simulink model "cascadeControl"  (R2020b)
settings: Solver=VariableStepAuto  StartTime=0.0  StopTime=40  RelTol=1e-3
values from neighbouring files (symbols this model uses):
  a_max = 4    [initialization.m]
  condtheta = 0    [initialization.m]
  condx = 0.0001    [initialization.m]
  condy = 0    [initialization.m]
  k = 1    [initialization.m]
  k_a = 2    [initialization.m]
  k_obsx = 5    [initialization.m]
  k_obsy = 5    [initialization.m]
  omega_max = 0.1    [initialization.m]
  slope_circ = 0.2    [initialization.m]
  v_max = 0.5    [initialization.m]
  v_square = 0.2    [initialization.m]
undefined symbols (not defined in the file or in its folder): sat_om
libraries: simulink x2
settings Model: Creator=adelina  LastModifiedBy=adelina
settings SolverCC: ZeroCrossAlgorithm=Adaptive
settings DebuggingCC: IgnoredZcDiagnostic=none

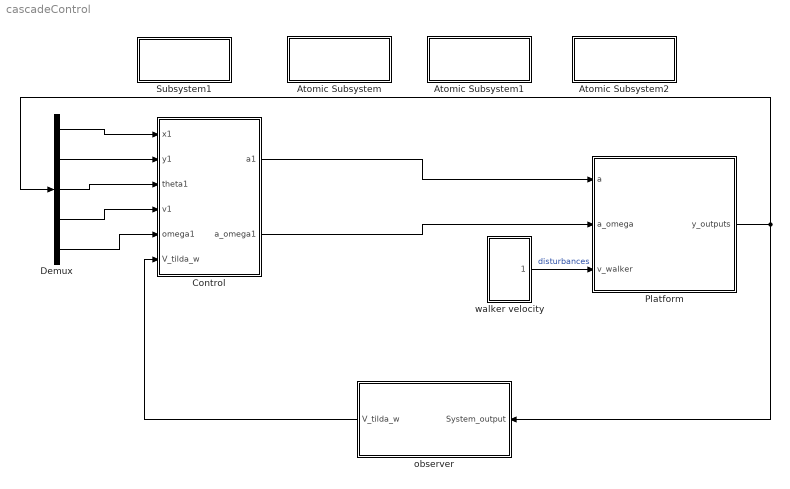
== system cascadeControl ==
  Atomic Subsystem : Subsystem  TreatAsAtomicUnit=on
      settings: OpenFcn=animation
      mask Display: disp('animation')
  Atomic Subsystem1 : Subsystem  TreatAsAtomicUnit=on
      settings: OpenFcn=plot_inputs
      mask Display: disp('plot inputs')
  Atomic Subsystem2 : Subsystem  TreatAsAtomicUnit=on
      settings: OpenFcn=plot_states
      mask Display: disp('plot states')
  Control : Subsystem
  Demux : Demux  Outputs=5
  Platform : Subsystem
  Subsystem1 : Subsystem
      settings: OpenFcn=plot_trajectory_frames
      mask Display: disp('plots')
  observer : Subsystem
  walker velocity : Subsystem
  wires:
  walker velocity/1(v_walker) -> Platform/3(v_walker)  "disturbances"
  Platform/1(y_outputs) -> observer/1(System_output), Demux/1
  Control/1(a1) -> Platform/1(a)
  Control/2(a_omega1) -> Platform/2(a_omega)
  Demux/3 -> Control/3(theta1)
  Demux/2 -> Control/2(y1)
  Demux/1 -> Control/1(x1)
  Demux/4 -> Control/4(v1)
  Demux/5 -> Control/5(omega1)
  observer/1(V_tilda_w) -> Control/6(V_tilda_w)

== system cascadeControl/Atomic Subsystem ==

== system cascadeControl/Atomic Subsystem1 ==

== system cascadeControl/Atomic Subsystem2 ==

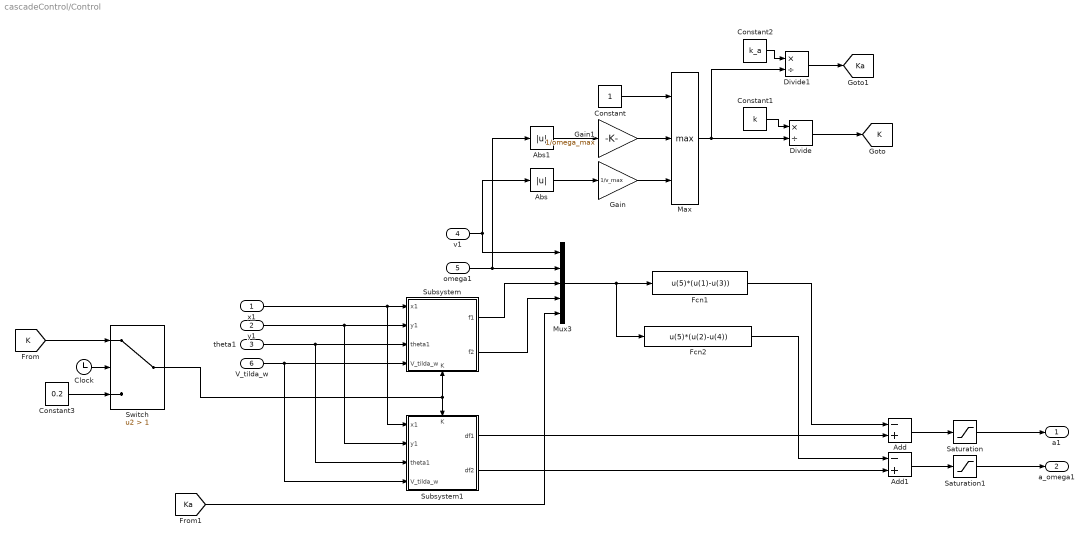
== system cascadeControl/Control ==
  x1 : Inport
  y1 : Inport  Port=2
  theta1 : Inport  Port=3
  v1 : Inport  Port=4
  omega1 : Inport  Port=5
  V_tilda_w : Inport  Port=6
  Abs : Abs
  Abs1 : Abs
  Add : Sum  Inputs=-+
  Add1 : Sum  Inputs=-+
  Clock : Clock
  Constant : Constant
  Constant1 : Constant  Value=k
  Constant2 : Constant  Value=k_a
  Constant3 : Constant  Value=0.2
  Divide : Product  Inputs=*/  RndMeth=Zero  SaturateOnIntegerOverflow=on
  Divide1 : Product  Inputs=*/  RndMeth=Zero  SaturateOnIntegerOverflow=on
  Fcn1 : Fcn  Expr=u(5)*(u(1)-u(3))
  Fcn2 : Fcn  Expr=u(5)*(u(2)-u(4))
  Gain : Gain  Gain=1/v_max
  Gain1 : Gain  Gain=1/omega_max
  Max : MinMax  Function=max  Inputs=3
  Mux3 : Mux  Inputs=5
  Saturation : Saturate  UpperLimit=a_max  LowerLimit=-a_max  ZeroCross=off
  Saturation1 : Saturate  UpperLimit=a_max  LowerLimit=-a_max  ZeroCross=off
  Subsystem : Subsystem
      settings: PortSchema="{\"entries\":[{\"content\":{\"sides\":[{\"content\":{\"connectorIds\":[\"In1\",\"In2\",\"In3\",\"In4\"]},\"type\":\"ConnectorPlacement.EquallySpacedRectSide\",\"uuid\":\"98a92254-b9ad-4bc0-80a4-de031a5e2866\"},{\"content\":{\"connectorIds\":[\"Out1\",\"Out2\"],\"side\":\"RIGHT\"},\"type\":\"ConnectorPlacement.EquallySpacedRectSide\",\"uuid\":\"e0692c06-8f6c-4190-87dc-563178f83e51\"},{\"content\":{\"connectorIds\":[],\"side\":\"TOP\"},\"type\":\"ConnectorPlacement.EquallySpacedRectSide\",\"uuid\":\"24e54c67-c633-4464-84bd-e02cec2cb8a7\"},{\"content\":{\"connectorIds\":[\"In5\"],\"side\":\"BOTTOM\"},\"type\":\"ConnectorPlacement.EquallySpacedRectSide\",\"uuid\":\"19ff3774-67e6-4579-b3b2-94cf61eef82b\"},{\"content\":{\"connectorIds\":[],\"side\":\"HIDDEN\"},\"type\":\"ConnectorPlacement.EquallySpacedRectSide\",\"uuid\":\"6a6977b6-e148-496e-85eb-1bd9ad7285df\"}]},\"type\":\"ConnectorPlacement.EquallySpacedConnector\",\"uuid\":\"5663e86b-5163-4af1-b1c3-40fc09afe5cc\"}],\"packageUris\":[\"http://schema.mathworks.com/mf0/Connector/R2020b\"],\"version\":\"1.0\"}"
  Subsystem1 : Subsystem
      settings: PortSchema="{\"entries\":[{\"content\":{\"sides\":[{\"content\":{\"connectorIds\":[\"In1\",\"In2\",\"In3\",\"In4\"]},\"type\":\"ConnectorPlacement.EquallySpacedRectSide\",\"uuid\":\"98a92254-b9ad-4bc0-80a4-de031a5e2866\"},{\"content\":{\"connectorIds\":[\"Out1\",\"Out2\"],\"side\":\"RIGHT\"},\"type\":\"ConnectorPlacement.EquallySpacedRectSide\",\"uuid\":\"e0692c06-8f6c-4190-87dc-563178f83e51\"},{\"content\":{\"connectorIds\":[\"In5\"],\"side\":\"TOP\"},\"type\":\"ConnectorPlacement.EquallySpacedRectSide\",\"uuid\":\"24e54c67-c633-4464-84bd-e02cec2cb8a7\"},{\"content\":{\"connectorIds\":[],\"side\":\"HIDDEN\"},\"type\":\"ConnectorPlacement.EquallySpacedRectSide\",\"uuid\":\"6a6977b6-e148-496e-85eb-1bd9ad7285df\"}]},\"type\":\"ConnectorPlacement.EquallySpacedConnector\",\"uuid\":\"5663e86b-5163-4af1-b1c3-40fc09afe5cc\"}],\"packageUris\":[\"http://schema.mathworks.com/mf0/Connector/R2020b\"],\"version\":\"1.0\"}"
  Switch : Switch  Criteria=u2 > Threshold  Threshold=1
  a1 : Outport
  a_omega1 : Outport  Port=2
  tag scope: K=global, Ka=global
  wires:
  x1/1 -> Subsystem1/1(x1), Subsystem/1(x1)
  y1/1 -> Subsystem1/2(y1), Subsystem/2(y1)
  theta1/1 -> Subsystem1/3(theta1), Subsystem/3(theta1)
  Subsystem/1(f1) -> Mux3/3
  Subsystem/2(f2) -> Mux3/4
  Mux3/1 -> Fcn1/1, Fcn2/1
  Subsystem1/1(df1) -> Add/2
  Fcn1/1 -> Add/1
  Fcn2/1 -> Add1/1
  Subsystem1/2(df2) -> Add1/2
  v1/1 -> Mux3/1, Abs/1
  omega1/1 -> Abs1/1, Mux3/2
  V_tilda_w/1 -> Subsystem1/4(V_tilda_w), Subsystem/4(V_tilda_w)
  Abs/1 -> Gain/1
  Gain/1 -> Max/3
  Abs1/1 -> Gain1/1
  Gain1/1 -> Max/2
  Constant/1 -> Max/1
  Max/1 -> Divide/2, Divide1/2
  Constant1/1 -> Divide/1
  Divide/1 -> [K]
  Saturation1/1 -> a_omega1/1
  Add1/1 -> Saturation1/1
  Add/1 -> Saturation/1
  Saturation/1 -> a1/1
  [Ka] -> Mux3/5
  Constant2/1 -> Divide1/1
  Divide1/1 -> [Ka]
  [K] -> Switch/1
  Clock/1 -> Switch/2
  Constant3/1 -> Switch/3
  Switch/1 -> Subsystem/5(K), Subsystem1/5(K)

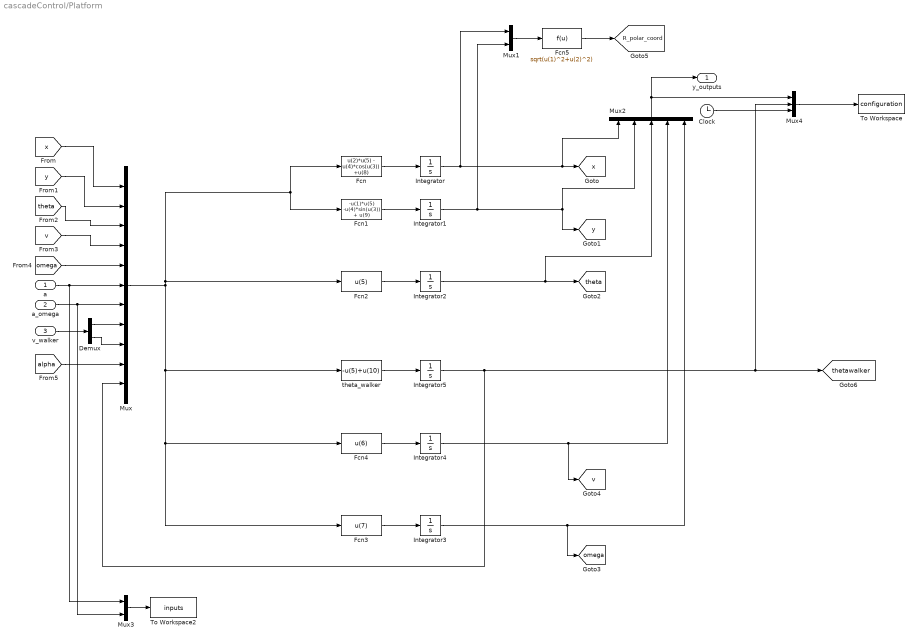
== system cascadeControl/Platform ==
  a : Inport
  a_omega : Inport  Port=2
  v_walker : Inport  Port=3
  Clock : Clock
  Demux : Demux  Outputs=2
  Fcn : Fcn  Expr=u(2)*u(5) - u(4)*cos(u(3)) +u(8)
  Fcn1 : Fcn  Expr=-u(1)*u(5) -u(4)*sin(u(3)) + u(9)
  Fcn2 : Fcn  Expr=u(5)
  Fcn3 : Fcn  Expr=u(7)
  Fcn4 : Fcn  Expr=u(6)
  Fcn5 : Fcn  Expr=sqrt(u(1)^2+u(2)^2)
  Integrator : Integrator  InitialCondition=condx
  Integrator1 : Integrator  InitialCondition=condy
  Integrator2 : Integrator  InitialCondition=condtheta
  Integrator3 : Integrator
  Integrator4 : Integrator
  Integrator5 : Integrator  InitialCondition=condtheta
  Mux : Mux  Inputs=11
  Mux1 : Mux  Inputs=2
  Mux2 : Mux  Inputs=5
  Mux3 : Mux  Inputs=2
  Mux4 : Mux  Inputs=3
  To Workspace : ToWorkspace  VariableName=configuration  SaveFormat=Structure With Time  SampleTime=-1
  To Workspace2 : ToWorkspace  VariableName=inputs  SaveFormat=Structure With Time  SampleTime=-1
  theta_walker : Fcn  Expr=-u(5)+u(10)
  y_outputs : Outport
  tag scope: R_polar_coord=global, omega=global, theta=global, thetawalker=global, v=global, x=global, y=global
  wires:
  Fcn2/1 -> Integrator2/1
  Integrator2/1 -> [theta], Mux2/3
  Fcn1/1 -> Integrator1/1
  [y] -> Mux/2
  [x] -> Mux/1
  a/1 -> Mux3/1, Mux/6
  Integrator1/1 -> Mux1/2, [y], Mux2/2
  [theta] -> Mux/3
  Integrator/1 -> Mux1/1, Mux2/1, [x]
  Fcn/1 -> Integrator/1
  a_omega/1 -> Mux3/2, Mux/7
  Mux2/1 -> y_outputs/1, Mux4/1
  [v] -> Mux/4
  [omega] -> Mux/5
  Integrator3/1 -> Mux2/5, [omega]
  Fcn3/1 -> Integrator3/1
  Integrator4/1 -> [v], Mux2/4
  Fcn4/1 -> Integrator4/1
  Mux1/1 -> Fcn5/1
  Fcn5/1 -> [R_polar_coord]
  Mux3/1 -> To Workspace2/1
  Clock/1 -> Mux4/3
  Mux4/1 -> To Workspace/1
  v_walker/1 -> Demux/1
  Demux/1 -> Mux/8
  Demux/2 -> Mux/9
  [alpha] -> Mux/10
  Mux/1 -> Fcn1/1, Fcn/1, Fcn2/1, theta_walker/1, Fcn3/1, Fcn4/1
  theta_walker/1 -> Integrator5/1
  Integrator5/1 -> Mux/11, [thetawalker], Mux4/2

== system cascadeControl/Subsystem1 ==

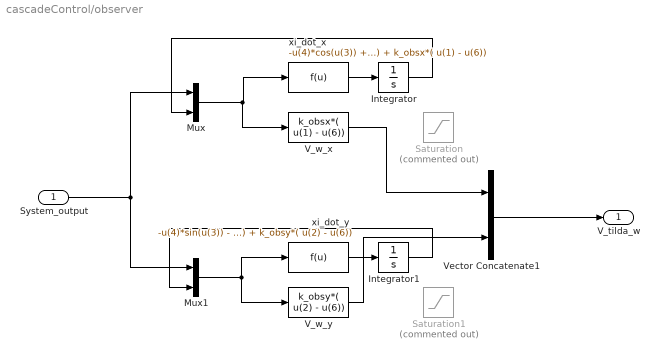
== system cascadeControl/observer ==
  System_output : Inport
  Integrator : Integrator  InitialCondition=condx
  Integrator1 : Integrator  InitialCondition=condy
  Mux : Mux  Inputs=2
  Mux1 : Mux  Inputs=2
  Saturation : Saturate  Commented=on
  Saturation1 : Saturate  Commented=on
  V_w_x : Fcn  Expr=k_obsx*( u(1) - u(6))
  V_w_y : Fcn  Expr=k_obsy*( u(2) - u(6))
  Vector Concatenate1 : Concatenate  Mode=Multidimensional array  ConcatenateDimension=2
  xi_dot_x : Fcn  Expr=-u(4)*cos(u(3)) + u(2)*u(5) + k_obsx*( u(1) - u(6))
  xi_dot_y : Fcn  Expr=-u(4)*sin(u(3)) - u(1)*u(5) + k_obsy*( u(2) - u(6))
  V_tilda_w : Outport
  wires:
  Mux/1 -> V_w_x/1, xi_dot_x/1
  Mux1/1 -> V_w_y/1, xi_dot_y/1
  System_output/1 -> Mux/1, Mux1/1
  Vector Concatenate1/1 -> V_tilda_w/1
  xi_dot_x/1 -> Integrator/1
  Integrator/1 -> Mux/2
  xi_dot_y/1 -> Integrator1/1
  Integrator1/1 -> Mux1/2
  V_w_y/1 -> Vector Concatenate1/2
  V_w_x/1 -> Vector Concatenate1/1

== system cascadeControl/walker velocity ==
  Circular path : Subsystem
  DocBlock : simulink/Model-Wide Utilities/DocBlock  DocumentType=Text
      content=|
      | Choose one of the trajectory by uncommenting and connecting with the output
  "Vx, Vy nonzero" : Subsystem  Commented=on
  square path : Subsystem  Commented=on
  v_walker : Outport
  wires:
  Circular path/1(v_walker) -> v_walker/1

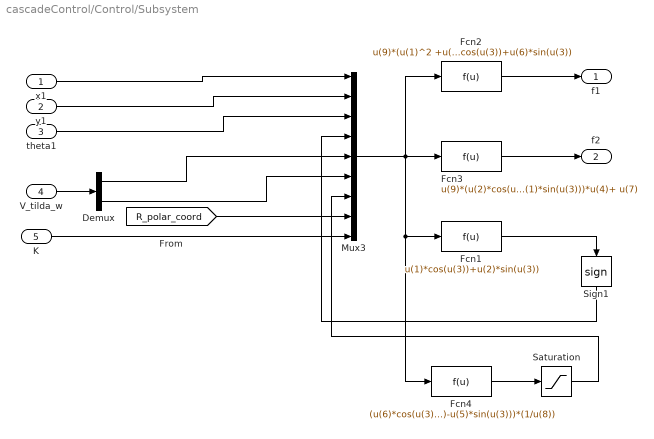
== system cascadeControl/Control/Subsystem ==
  x1 : Inport
  y1 : Inport  Port=2
  theta1 : Inport  Port=3
  V_tilda_w : Inport  Port=4
  K : Inport  Port=5
  Demux : Demux  Outputs=2
  Fcn1 : Fcn  Expr=u(1)*cos(u(3))+u(2)*sin(u(3))
  Fcn2 : Fcn  Expr=u(9)*(u(1)^2 +u(2)^2)*u(4)+u(5)*cos(u(3))+u(6)*sin(u(3))
  Fcn3 : Fcn  Expr=u(9)*(u(2)*cos(u(3))-u(1)*sin(u(3)))*u(4)+ u(7)
  Fcn4 : Fcn  Expr=(u(6)*cos(u(3))-u(5)*sin(u(3)))*(1/u(8))
  Mux3 : Mux  Inputs=9
  Saturation : Saturate  UpperLimit=sat_om  LowerLimit=-sat_om
  Sign1 : Signum  ZeroCross=off
  f1 : Outport
  f2 : Outport  Port=2
  wires:
  Sign1/1 -> Mux3/4
  y1/1 -> Mux3/2
  x1/1 -> Mux3/1
  theta1/1 -> Mux3/3
  Fcn1/1 -> Sign1/1
  Mux3/1 -> Fcn4/1, Fcn1/1, Fcn2/1, Fcn3/1
  Fcn2/1 -> f1/1
  Fcn3/1 -> f2/1
  V_tilda_w/1 -> Demux/1
  Demux/1 -> Mux3/5
  Demux/2 -> Mux3/6
  Fcn4/1 -> Saturation/1
  Saturation/1 -> Mux3/7
  [R_polar_coord] -> Mux3/8
  K/1 -> Mux3/9

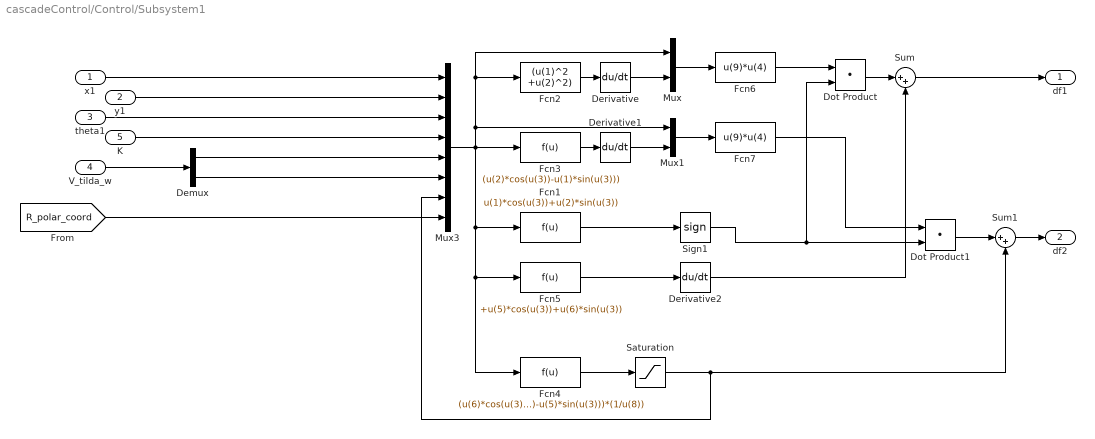
== system cascadeControl/Control/Subsystem1 ==
  x1 : Inport
  y1 : Inport  Port=2
  theta1 : Inport  Port=3
  V_tilda_w : Inport  Port=4
  K : Inport  Port=5
  Demux : Demux  Outputs=2
  Derivative : Derivative
  Derivative1 : Derivative
  Derivative2 : Derivative
  Dot Product : DotProduct  InputSameDT=on  OutDataTypeStr=Inherit: Inherit via internal rule
  Dot Product1 : DotProduct  InputSameDT=on  OutDataTypeStr=Inherit: Inherit via internal rule
  Fcn1 : Fcn  Expr=u(1)*cos(u(3))+u(2)*sin(u(3))
  Fcn2 : Fcn  Expr=(u(1)^2 +u(2)^2)
  Fcn3 : Fcn  Expr=(u(2)*cos(u(3))-u(1)*sin(u(3)))
  Fcn4 : Fcn  Expr=(u(6)*cos(u(3))-u(5)*sin(u(3)))*(1/u(8))
  Fcn5 : Fcn  Expr=+u(5)*cos(u(3))+u(6)*sin(u(3))
  Fcn6 : Fcn  Expr=u(9)*u(4)
  Fcn7 : Fcn  Expr=u(9)*u(4)
  Mux : Mux  Inputs=2
  Mux1 : Mux  Inputs=2
  Mux3 : Mux  Inputs=8
  Saturation : Saturate  UpperLimit=sat_om  LowerLimit=-sat_om
  Sign1 : Signum  ZeroCross=off
  Sum : Sum  Inputs=|++
  Sum1 : Sum  Inputs=|++
  df1 : Outport
  df2 : Outport  Port=2
  wires:
  y1/1 -> Mux3/2
  Fcn1/1 -> Sign1/1
  Mux3/1 -> Fcn3/1, Fcn1/1, Fcn5/1, Fcn4/1, Mux1/1, Fcn2/1, Mux/1
  theta1/1 -> Mux3/3
  Demux/1 -> Mux3/5
  x1/1 -> Mux3/1
  [R_polar_coord] -> Mux3/8
  Fcn4/1 -> Saturation/1
  Saturation/1 -> Sum1/2, Mux3/7
  V_tilda_w/1 -> Demux/1
  Demux/2 -> Mux3/6
  Fcn2/1 -> Derivative/1
  Fcn3/1 -> Derivative1/1
  Dot Product/1 -> Sum/1
  Fcn5/1 -> Derivative2/1
  Sum/1 -> df1/1
  Sum1/1 -> df2/1
  Derivative2/1 -> Sum/2
  Dot Product1/1 -> Sum1/1
  Sign1/1 -> Dot Product/2, Dot Product1/2
  K/1 -> Mux3/4
  Derivative/1 -> Mux/2
  Mux/1 -> Fcn6/1
  Fcn6/1 -> Dot Product/1
  Mux1/1 -> Fcn7/1
  Derivative1/1 -> Mux1/2
  Fcn7/1 -> Dot Product1/1

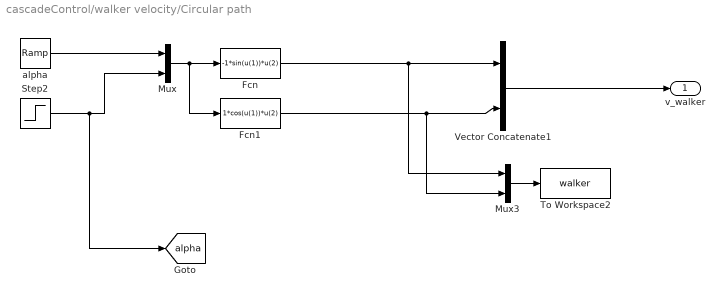
== system cascadeControl/walker velocity/Circular path ==
  Fcn : Fcn  Expr=-1*sin(u(1))*u(2)
  Fcn1 : Fcn  Expr=1*cos(u(1))*u(2)
  Mux : Mux  Inputs=2
  Mux3 : Mux  Inputs=2
  Step2 : Step  After=slope_circ  SampleTime=0
  To Workspace2 : ToWorkspace  VariableName=walker  SaveFormat=Structure With Time  SampleTime=-1
  Vector Concatenate1 : Concatenate  Mode=Multidimensional array  ConcatenateDimension=2
  alpha : simulink/Sources/Ramp  slope=slope_circ  start=1  InitialOutput=0
  v_walker : Outport
  tag scope: alpha=global
  wires:
  alpha/1 -> Mux/1
  Fcn1/1 -> Vector Concatenate1/2, Mux3/2
  Fcn/1 -> Mux3/1, Vector Concatenate1/1
  Vector Concatenate1/1 -> v_walker/1
  Mux3/1 -> To Workspace2/1
  Mux/1 -> Fcn1/1, Fcn/1
  Step2/1 -> [alpha], Mux/2

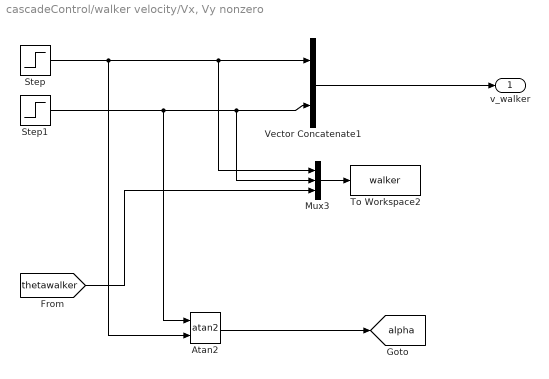
== system cascadeControl/walker velocity/Vx, Vy nonzero ==
  Atan2 : Trigonometry  Operator=atan2
  Mux3 : Mux  Inputs=3
  Step : Step  Time=2  After=0  SampleTime=0
  Step1 : Step  Time=0  After=0  SampleTime=0
  To Workspace2 : ToWorkspace  VariableName=walker  SaveFormat=Structure With Time  SampleTime=-1
  Vector Concatenate1 : Concatenate  Mode=Multidimensional array  ConcatenateDimension=2
  v_walker : Outport
  tag scope: alpha=global
  wires:
  Vector Concatenate1/1 -> v_walker/1
  Mux3/1 -> To Workspace2/1
  Step/1 -> Atan2/2, Mux3/1, Vector Concatenate1/1
  Step1/1 -> Atan2/1, Vector Concatenate1/2, Mux3/2
  [thetawalker] -> Mux3/3
  Atan2/1 -> [alpha]

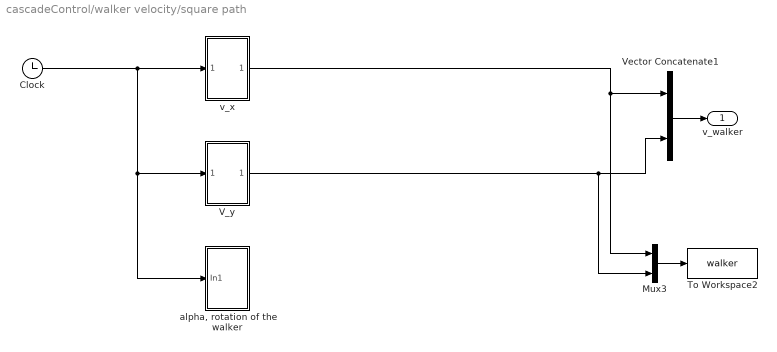
== system cascadeControl/walker velocity/square path ==
  Clock : Clock
  Mux3 : Mux  Inputs=2
  To Workspace2 : ToWorkspace  VariableName=walker  SaveFormat=Structure With Time  SampleTime=-1
  V_y : Subsystem
  Vector Concatenate1 : Concatenate  Mode=Multidimensional array  ConcatenateDimension=2
  "alpha, rotation of the walker" : Subsystem
  v_x : Subsystem
  v_walker : Outport
  wires:
  Vector Concatenate1/1 -> v_walker/1
  Mux3/1 -> To Workspace2/1
  Clock/1 -> v_x/1(In1), "alpha, rotation of the walker"/1(In1), V_y/1(In1)
  V_y/1(Out1) -> Mux3/2, Vector Concatenate1/2
  v_x/1(Out1) -> Mux3/1, Vector Concatenate1/1

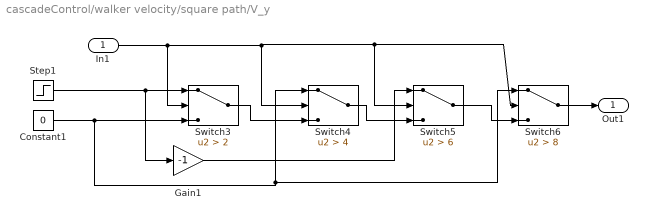
== system cascadeControl/walker velocity/square path/V_y ==
  In1 : Inport
  Constant1 : Constant  Value=0
  Gain1 : Gain  Gain=-1
  Step1 : Step  Time=0  After=v_square  SampleTime=0
  Switch3 : Switch  Criteria=u2 > Threshold  Threshold=2
  Switch4 : Switch  Criteria=u2 > Threshold  Threshold=4
  Switch5 : Switch  Criteria=u2 > Threshold  Threshold=6
  Switch6 : Switch  Criteria=u2 > Threshold  Threshold=8
  Out1 : Outport
  wires:
  Step1/1 -> Gain1/1, Switch3/1
  Switch6/1 -> Out1/1
  In1/1 -> Switch3/2, Switch5/2, Switch6/2, Switch4/2
  Switch5/1 -> Switch6/3
  Switch3/1 -> Switch4/3
  Constant1/1 -> Switch6/1, Switch4/1, Switch3/3
  Switch4/1 -> Switch5/3
  Gain1/1 -> Switch5/1

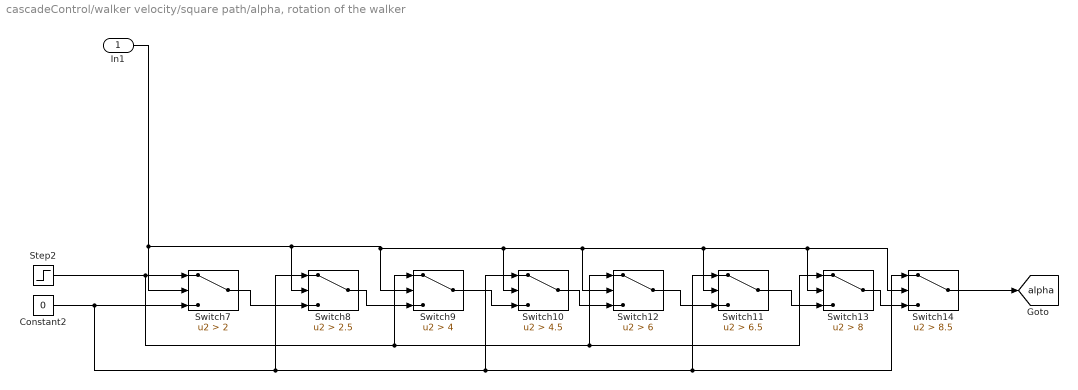
== system cascadeControl/walker velocity/square path/alpha, rotation of the walker ==
  In1 : Inport
  Constant2 : Constant  Value=0
  Step2 : Step  Time=0  After=pi  SampleTime=0
  Switch10 : Switch  Criteria=u2 > Threshold  Threshold=4.5
  Switch11 : Switch  Criteria=u2 > Threshold  Threshold=6.5
  Switch12 : Switch  Criteria=u2 > Threshold  Threshold=6
  Switch13 : Switch  Criteria=u2 > Threshold  Threshold=8
  Switch14 : Switch  Criteria=u2 > Threshold  Threshold=8.5
  Switch7 : Switch  Criteria=u2 > Threshold  Threshold=2
  Switch8 : Switch  Criteria=u2 > Threshold  Threshold=2.5
  Switch9 : Switch  Criteria=u2 > Threshold  Threshold=4
  tag scope: alpha=global
  wires:
  Switch11/1 -> Switch13/3
  Switch13/1 -> Switch14/3
  Switch14/1 -> [alpha]
  In1/1 -> Switch8/2, Switch12/2, Switch14/2, Switch13/2, Switch11/2, Switch10/2, Switch9/2, Switch7/2
  Switch9/1 -> Switch10/3
  Switch8/1 -> Switch9/3
  Switch10/1 -> Switch12/3
  Switch7/1 -> Switch8/3
  Step2/1 -> Switch9/1, Switch13/1, Switch12/1, Switch7/1
  Constant2/1 -> Switch8/1, Switch10/1, Switch11/1, Switch14/1, Switch7/3
  Switch12/1 -> Switch11/3

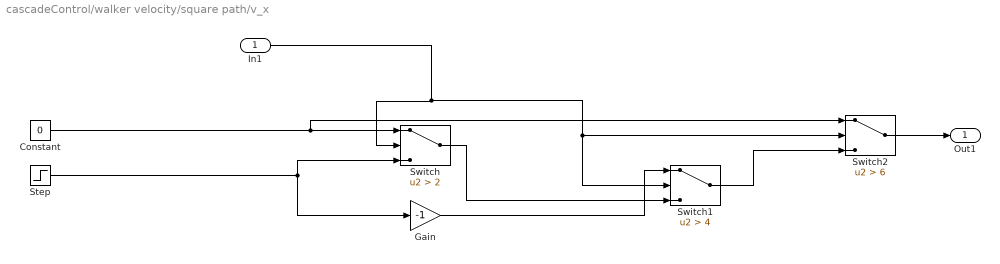
== system cascadeControl/walker velocity/square path/v_x ==
  In1 : Inport
  Constant : Constant  Value=0
  Gain : Gain  Gain=-1
  Step : Step  Time=0  After=v_square  SampleTime=0
  Switch : Switch  Criteria=u2 > Threshold  Threshold=2
  Switch1 : Switch  Criteria=u2 > Threshold  Threshold=4
  Switch2 : Switch  Criteria=u2 > Threshold  Threshold=6
  Out1 : Outport
  wires:
  Switch1/1 -> Switch2/3
  In1/1 -> Switch/2, Switch1/2, Switch2/2
  Gain/1 -> Switch1/1
  Switch/1 -> Switch1/3
  Step/1 -> Gain/1, Switch/3
  Constant/1 -> Switch2/1, Switch/1
  Switch2/1 -> Out1/1
